simulink model "AeroSFunctiontest2"  (R2021a)
settings: Solver=VariableStepAuto  StartTime=0.0  StopTime=10.0  RelTol=1e-3
settings Model: Creator=siddh  LastModifiedBy=siddh

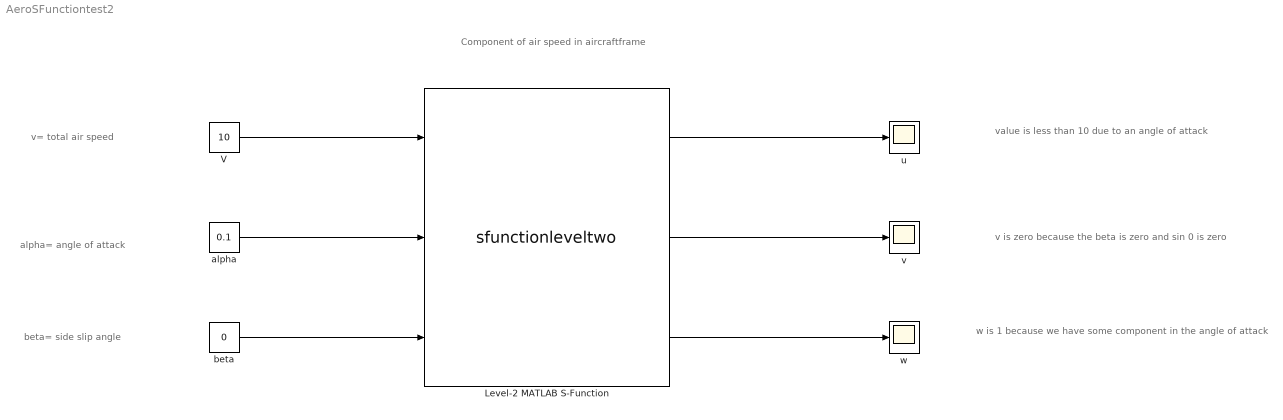
== system AeroSFunctiontest2 ==
  note: beta= side slip angle
  note: alpha= angle of attack
  note: v= total air speed
  note: Component of air speed in aircraftframe
  note: w is 1 because we have some component in the angle of attack
  note: v is zero because the beta is zero and sin 0 is zero
  note: value is less than 10 due to an angle of attack
  Level-2 MATLAB S-Function : M-S-Function  FunctionName=sfunctionleveltwo
  V : Constant  Value=10
  alpha : Constant  Value=0.1
  beta : Constant  Value=0
  u : Scope
  v : Scope
  w : Scope
  wires:
  V/1 -> Level-2 MATLAB S-Function/1
  alpha/1 -> Level-2 MATLAB S-Function/2
  beta/1 -> Level-2 MATLAB S-Function/3
  Level-2 MATLAB S-Function/1 -> u/1
  Level-2 MATLAB S-Function/2 -> v/1
  Level-2 MATLAB S-Function/3 -> w/1
